simulink model "test"  (R2024b)
settings: Solver=FixedStepAuto  StartTime=0.0  StopTime=inf  FixedStep=0.01  RelTol=1e-3
undefined symbols (not defined in the file): DiscIntNeverNeededParam, LF
libraries: instrumentseriallib x11
settings Model: Creator=USER  LastModifiedBy=USER
settings OptimizationCC: DefaultParameterBehavior=Inlined  EnhancedBackFolding=on  PassReuseOutputArgsAs=Individual arguments  ZeroExternalMemoryAtStartup=off  ZeroInternalMemoryAtStartup=off  OptimizeBlockOrder=speed  DifferentSizesBufferReuse=on  OptimizationCustomize=off  EfficientTunableParamExpr=on
settings DebuggingCC: ParameterTunabilityLossMsg=error
settings SFSimCC: MATLABDynamicMemAlloc=off
settings RTWCC: Description=Embedded Coder  SystemTargetFile=ert.tlc  GenCodeOnly=on  TemplateMakefile=ert_default_tmf
settings CodeAppCC: ForceParamTrailComments=on  IgnoreCustomStorageClasses=off  OperatorAnnotations=on  SimulinkDataObjDesc=on  SFDataObjDesc=on  InsertBlockDesc=on
settings ERTTargetCC: TargetLangStandard=C99 (ISO)  GenerateSampleERTMain=on  ERTCustomFileTemplate=example_file_process.tlc

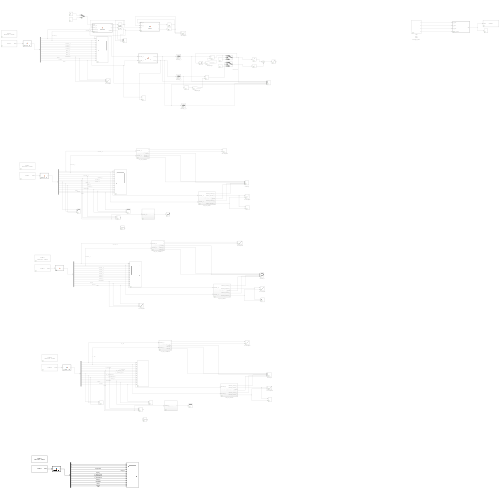
[thumbnail: Simulink's stored preview of the top-level diagram]
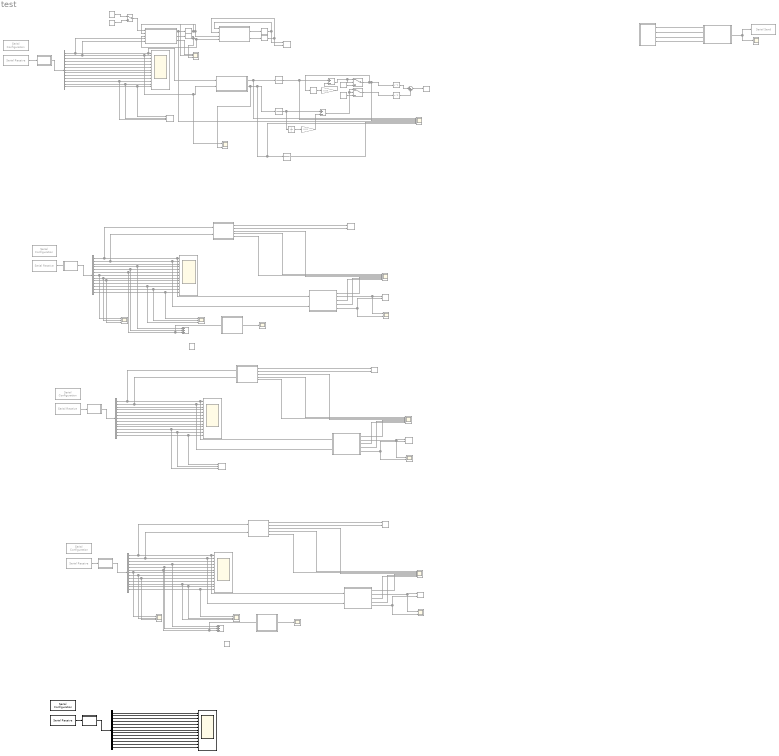
== system test ==
  1:Kp 2:Ki 3:Kd 4:target_pwm : Subsystem  Commented=on  mask{P_gain=1.0, I_gain=0.1, D_gain=0, PWM_speed=2000}
      mask prompts: P_gain "P gain"; I_gain "I gain"; D_gain "D gain"; PWM_speed "PWM Speed"
      mask DialogControl ParameterGroupVar Prompt: 파라미터
  Add : Sum  Commented=on  Inputs=+++
  Add1 : Sum  Commented=on  Inputs=+-
  Add2 : Sum  Commented=on  Inputs=+-
  Add3 : Sum  Commented=on  Inputs=+++
  Atan1 : Trigonometry  Commented=on  Operator=atan2
  Atan2 : Trigonometry  Commented=on  Operator=atan2
  Constant : Constant  Commented=on  Value=0
  Constant1 : Constant  Commented=on
  Constant3 : Constant  Commented=on  Value=0
  Constant4 : Constant  Commented=on  Value=0
  Demux{,1..3} (4 alike) : Demux  Commented=on  Outputs=13
  Demux4 : Demux  Outputs=13
  MATLAB Function : MATLAB Function  Commented=on  TreatAsAtomicUnit=on
  MATLAB Function1 : MATLAB Function  Commented=on  TreatAsAtomicUnit=on
  MATLAB Function2 : MATLAB Function  Commented=on  TreatAsAtomicUnit=on
  MATLAB Function3 : MATLAB Function  Commented=on  TreatAsAtomicUnit=on
  MATLAB Function4 : MATLAB Function  Commented=on  TreatAsAtomicUnit=on
  MATLAB Function5 : MATLAB Function  Commented=on  TreatAsAtomicUnit=on
  MATLAB Function6 : MATLAB Function  Commented=on  TreatAsAtomicUnit=on
  MATLAB Function7 : MATLAB Function  Commented=on  TreatAsAtomicUnit=on
  MATLAB Function8 : MATLAB Function  TreatAsAtomicUnit=on
  Manual Switch : ManualSwitch  Commented=on
  Memory{,1..4} (5 alike) : Memory  Commented=on
  Scope{,9..10,12,16} (5 alike) : Scope  Commented=on  NumInputPorts=3
  Scope1 : Scope  Commented=on
  Scope11 : Scope  Commented=on
  Scope13 : Scope  Commented=on
  Scope{4..5,7,14} (4 alike) : Scope  Commented=on  NumInputPorts=2
  Scope{2,6,8,15} (4 alike) : Scope  Commented=on  NumInputPorts=13
  Scope20 : Scope  NumInputPorts=13
  Scope3 : Scope  Commented=on  NumInputPorts=6
  Serial Configuration : instrumentseriallib/Serial Configuration  Priority=-200000  Commented=on  PortSel=COM17  Port=COM17  ComPort=COM17  BaudRate=115200  DataBits=8  Parity=none  StopBits=1  ByteOrder=big-endian  FlowControl=none  Timeout=1  SimulateUsing=Interpreted execution  BlockInModel=on  aMode=1
  Serial Configuration1 : instrumentseriallib/Serial Configuration  Priority=-200000  Commented=on  PortSel=COM17  Port=COM17  ComPort=COM17  BaudRate=115200  DataBits=8  Parity=none  StopBits=1  ByteOrder=big-endian  FlowControl=none  Timeout=1  SimulateUsing=Interpreted execution  BlockInModel=on  aMode=1
  Serial Configuration2 : instrumentseriallib/Serial Configuration  Priority=-200000  Commented=on  PortSel=COM17  Port=COM17  ComPort=COM17  BaudRate=115200  DataBits=8  Parity=none  StopBits=1  ByteOrder=big-endian  FlowControl=none  Timeout=1  SimulateUsing=Interpreted execution  BlockInModel=on  aMode=1
  Serial Configuration3 : instrumentseriallib/Serial Configuration  Priority=-200000  Commented=on  PortSel=COM19  Port=COM19  ComPort=COM19  BaudRate=115200  DataBits=8  Parity=none  StopBits=1  ByteOrder=big-endian  FlowControl=none  Timeout=1  SimulateUsing=Interpreted execution  BlockInModel=on  aMode=1
  Serial Configuration4 : instrumentseriallib/Serial Configuration  Priority=-200000  PortSel=COM19  Port=COM19  ComPort=COM19  BaudRate=115200  DataBits=8  Parity=none  StopBits=1  ByteOrder=big-endian  FlowControl=none  Timeout=1  SimulateUsing=Interpreted execution  BlockInModel=on  aMode=1
  Serial Receive : instrumentseriallib/Serial Receive  Priority=1  Commented=on  PortSel=COM17  Port=COM17  ComPort=COM17  DataType=uint8  SaveDataType=uint8  ToggleHeader=off  Header=[]  ToggleDataSize=on  DataSize=[1 130]  ToggleTerminator=on  Terminator=LF ('\n')  CustomTerminator=[]  InputFormat=Column major  EnableBlockingMode=on  ActionDataUnavailable=Output last received value  ActionWhenDataUnavailable=Output last received value  CustomValue=0  SampleTime=0.01  SimulateUsing=Interpreted execution  BlockInModel=on  aMode=1
  Serial Receive1 : instrumentseriallib/Serial Receive  Priority=1  Commented=on  PortSel=COM17  Port=COM17  ComPort=COM17  DataType=uint8  SaveDataType=uint8  ToggleHeader=off  Header=[]  ToggleDataSize=on  DataSize=[1 130]  ToggleTerminator=on  Terminator=LF ('\n')  CustomTerminator=[]  InputFormat=Column major  EnableBlockingMode=on  ActionDataUnavailable=Output last received value  ActionWhenDataUnavailable=Output last received value  CustomValue=0  SampleTime=0.01  SimulateUsing=Interpreted execution  BlockInModel=on  aMode=1
  Serial Receive2 : instrumentseriallib/Serial Receive  Priority=1  Commented=on  PortSel=COM17  Port=COM17  ComPort=COM17  DataType=uint8  SaveDataType=uint8  ToggleHeader=off  Header=[]  ToggleDataSize=on  DataSize=[1 130]  ToggleTerminator=on  Terminator=LF ('\n')  CustomTerminator=[]  InputFormat=Column major  EnableBlockingMode=on  ActionDataUnavailable=Output last received value  ActionWhenDataUnavailable=Output last received value  CustomValue=0  SampleTime=0.01  SimulateUsing=Interpreted execution  BlockInModel=on  aMode=1
  Serial Receive3 : instrumentseriallib/Serial Receive  Priority=1  Commented=on  PortSel=COM19  Port=COM19  ComPort=COM19  DataType=uint8  SaveDataType=uint8  ToggleHeader=off  Header=[]  ToggleDataSize=on  DataSize=[1 130]  ToggleTerminator=on  Terminator=LF ('\n')  CustomTerminator=[]  InputFormat=Column major  EnableBlockingMode=on  ActionDataUnavailable=Output last received value  ActionWhenDataUnavailable=Output last received value  CustomValue=0  SampleTime=0.01  SimulateUsing=Interpreted execution  BlockInModel=on  aMode=1
  Serial Receive4 : instrumentseriallib/Serial Receive  Priority=1  PortSel=COM19  Port=COM19  ComPort=COM19  DataType=uint8  SaveDataType=uint8  ToggleHeader=off  Header=[]  ToggleDataSize=on  DataSize=[1 130]  ToggleTerminator=on  Terminator=LF ('\n')  CustomTerminator=[]  InputFormat=Column major  EnableBlockingMode=on  ActionDataUnavailable=Output last received value  ActionWhenDataUnavailable=Output last received value  CustomValue=0  SampleTime=0.01  SimulateUsing=Interpreted execution  BlockInModel=on  aMode=1
  Serial Send : instrumentseriallib/Serial Send  Priority=1  Commented=on  PortSel=COM17  Port=COM17  ComPort=COM17  Header=[]  Terminator=<none>  CustomTerminator=[]  EnableBlockingMode=on  SimulateUsing=Interpreted execution  BlockInModel=on  aMode=1
  Sqrt : Sqrt  Commented=on
  Square : Math  Commented=on  Operator=square
  Square1 : Math  Commented=on  Operator=square
  Subsystem : Subsystem  Commented=on
  Subsystem1 : Subsystem  Commented=on
  Sum : Sum  Commented=on  Inputs=|++
  Switch : Switch  Commented=on  Criteria=u2 > Threshold  SaturateOnIntegerOverflow=off  InputSameDT=off
  Switch1 : Switch  Commented=on  Criteria=u2 > Threshold  SaturateOnIntegerOverflow=off  InputSameDT=off
  Unit Delay1 : UnitDelay  Commented=on  SampleTime=-1  HasFrameUpgradeWarning=on
  XY Graph{,1,5..7} (5 alike) : Record  Commented=on  FileSettingsInternal="{\"entries\":[{\"content\":{\"excelSettings\":{\"content\":{},\"type\":\"Streamout.ExcelSettings\"}},\"type\":\"Streamout.FileSettingStorage\",\"uuid\":\"\"}],\"packageUris\":[\"http:\\/\\/schema.mathworks.com\\/mf0\\/streamout_blocks\\/R2020a\"],\"version\":\"1.0\"}"  Layout=[1 1]  SignalsInternal="{\"entries\":[{\"content\":{},\"type\":\"RecordBlkView.InputSignals\",\"uuid\":\"\"}],\"packageUris\":[\"http:\\/\\/schema.mathworks.com\\/mf0\\/streamout_blocks\\/R2020a\"],\"version\":\"1.0\"}"  VisualizationBindings="{\"xyplotplugin\":{\"info\":[{\"series\":[],\"subplotID\":1}]}}"  CompatibilityTag=XY
  XY Graph2 : Record  Commented=on  FileSettingsInternal="{\"entries\":[{\"content\":{\"excelSettings\":{\"content\":{},\"type\":\"Streamout.ExcelSettings\"}},\"type\":\"Streamout.FileSettingStorage\",\"uuid\":\"\"}],\"packageUris\":[\"http:\\/\\/schema.mathworks.com\\/mf0\\/streamout_blocks\\/R2020a\"],\"version\":\"1.0\"}"  Layout=[1 1]  SignalsInternal="{\"entries\":[{\"content\":{\"signals\":[{\"content\":{\"blockPath\":[],\"dimensions\":[1],\"domain\":\"\",\"lineColor\":\"#edb120\",\"lineWidth\":2,\"port\":1,\"signalID\":1,\"signalName\":\"vel_loc_nofilter:1\"},\"type\":\"RecordBlkView.Signal\",\"uuid\":\"\"},{\"content\":{\"blockPath\":[],\"dimensions\":[1],\"domain\":\"\",\"lineColor\":\"#7e2f8e\",\"lineWidth\":2,\"port\":2,\"signalID\":2,\"signalName\":\"vel_loc_nofilter:2\"},\"type\":\"RecordBlkView.Signal\",\"uuid\":\"\"}]},\"type\":\"RecordBlkView.InputSignals\",\"uuid\":\"\"}],\"packageUris\":[\"http:\\/\\/schema.mathworks.com\\/mf0\\/streamout_blocks\\/R2020a\"],\"version\":\"1.0\"}"  VisualizationBindings="{\"xyplotplugin\":{\"info\":[{\"series\":[],\"subplotID\":1}]}}"  CompatibilityTag=XY
  XY Graph3 : Record  Commented=on  FileSettingsInternal="{\"entries\":[{\"content\":{\"excelSettings\":{\"content\":{},\"type\":\"Streamout.ExcelSettings\"}},\"type\":\"Streamout.FileSettingStorage\",\"uuid\":\"\"}],\"packageUris\":[\"http:\\/\\/schema.mathworks.com\\/mf0\\/streamout_blocks\\/R2020a\"],\"version\":\"1.0\"}"  Layout=[1 1]  SignalsInternal="{\"entries\":[{\"content\":{\"signals\":[{\"content\":{\"blockPath\":[],\"dimensions\":[1],\"domain\":\"\",\"lineColor\":\"#64d413\",\"lineWidth\":2,\"port\":1,\"signalID\":1,\"signalName\":\"vel_loc_nofilter2:1\"},\"type\":\"RecordBlkView.Signal\",\"uuid\":\"\"},{\"content\":{\"blockPath\":[],\"dimensions\":[1],\"domain\":\"\",\"lineColor\":\"#ff13a6\",\"lineWidth\":2,\"port\":2,\"signalID\":2,\"signalName\":\"vel_loc_nofilter2:2\"},\"type\":\"RecordBlkView.Signal\",\"uuid\":\"\"}]},\"type\":\"RecordBlkView.InputSignals\",\"uuid\":\"\"}],\"packageUris\":[\"http:\\/\\/schema.mathworks.com\\/mf0\\/streamout_blocks\\/R2020a\"],\"version\":\"1.0\"}"  VisualizationBindings="{\"xyplotplugin\":{\"info\":[{\"series\":[],\"subplotID\":1}]}}"  CompatibilityTag=XY
  XY Graph4 : Record  Commented=on  FileSettingsInternal="{\"entries\":[{\"content\":{\"excelSettings\":{\"content\":{},\"type\":\"Streamout.ExcelSettings\"}},\"type\":\"Streamout.FileSettingStorage\",\"uuid\":\"\"}],\"packageUris\":[\"http:\\/\\/schema.mathworks.com\\/mf0\\/streamout_blocks\\/R2020a\"],\"version\":\"1.0\"}"  Layout=[1 1]  SignalsInternal="{\"entries\":[{\"content\":{\"signals\":[{\"content\":{\"blockPath\":[],\"dimensions\":[1],\"domain\":\"\",\"lineColor\":\"#77ac30\",\"lineWidth\":2,\"port\":1,\"signalID\":1,\"signalName\":\"vel_loc_Filter:2\"},\"type\":\"RecordBlkView.Signal\",\"uuid\":\"\"},{\"content\":{\"blockPath\":[],\"dimensions\":[1],\"domain\":\"\",\"lineColor\":\"#4dbeee\",\"lineWidth\":2,\"port\":2,\"signalID\":2,\"signalName\":\"vel_loc_Filter:5\"},\"type\":\"RecordBlkView.Signal\",\"uuid\":\"\"}]},\"type\":\"RecordBlkView.InputSignals\",\"uuid\":\"\"}],\"packageUris\":[\"http:\\/\\/schema.mathworks.com\\/mf0\\/streamout_blocks\\/R2020a\"],\"version\":\"1.0\"}"  VisualizationBindings="{\"xyplotplugin\":{\"info\":[{\"series\":[],\"subplotID\":1}]}}"  CompatibilityTag=XY
  XY Graph8 : Record  Commented=on  FileSettingsInternal="{\"entries\":[{\"content\":{\"excelSettings\":{\"content\":{},\"type\":\"Streamout.ExcelSettings\"}},\"type\":\"Streamout.FileSettingStorage\",\"uuid\":\"\"}],\"packageUris\":[\"http:\\/\\/schema.mathworks.com\\/mf0\\/streamout_blocks\\/R2020a\"],\"version\":\"1.0\"}"  Layout=[1 1]  SignalsInternal="{\"entries\":[{\"content\":{\"signals\":[{\"content\":{\"blockPath\":[],\"dimensions\":[1],\"domain\":\"\",\"lineColor\":\"#fe330a\",\"lineWidth\":2,\"port\":1,\"signalID\":1,\"signalName\":\"vel_loc_Filter2:2\"},\"type\":\"RecordBlkView.Signal\",\"uuid\":\"\"},{\"content\":{\"blockPath\":[],\"dimensions\":[1],\"domain\":\"\",\"lineColor\":\"#22b573\",\"lineWidth\":2,\"port\":2,\"signalID\":2,\"signalName\":\"vel_loc_Filter2:5\"},\"type\":\"RecordBlkView.Signal\",\"uuid\":\"\"}]},\"type\":\"RecordBlkView.InputSignals\",\"uuid\":\"\"}],\"packageUris\":[\"http:\\/\\/schema.mathworks.com\\/mf0\\/streamout_blocks\\/R2020a\"],\"version\":\"1.0\"}"  VisualizationBindings="{\"xyplotplugin\":{\"info\":[{\"series\":[],\"subplotID\":1}]}}"  CompatibilityTag=XY
  damping1 : Gain  Commented=on  Gain=0.05
  damping2 : Gain  Commented=on  Gain=0.01
  vel_loc_Filter : Subsystem  Commented=on
  vel_loc_Filter1 : Subsystem  Commented=on
  vel_loc_Filter2 : Subsystem  Commented=on
  vel_loc_nofilter : Subsystem  Commented=on
  vel_loc_nofilter1 : Subsystem  Commented=on
  vel_loc_nofilter2 : Subsystem  Commented=on
  velocity : Scope  Commented=on  NumInputPorts=6
  velocity1 : Scope  Commented=on  NumInputPorts=6
  velocity2 : Scope  Commented=on  NumInputPorts=6
  velocity_x : DiscreteIntegrator  Commented=on  IntegratorMethod=Integration: Backward Euler  gainval=0.01  InitialCondition=0.001  SampleTime=0.01  ICPrevOutput=DiscIntNeverNeededParam  ICPrevScaledInput=DiscIntNeverNeededParam
  velocity_y : DiscreteIntegrator  Commented=on  IntegratorMethod=Integration: Backward Euler  gainval=0.01  SampleTime=0.01  ICPrevOutput=DiscIntNeverNeededParam  ICPrevScaledInput=DiscIntNeverNeededParam
  velocity_y1 : DiscreteIntegrator  Commented=on  IntegratorMethod=Integration: Backward Euler  gainval=0.01  InitialCondition=0.001  SampleTime=0.01  ICPrevOutput=DiscIntNeverNeededParam  ICPrevScaledInput=DiscIntNeverNeededParam
  wires:
  Serial Receive/1 -> MATLAB Function/1(u)
  1:Kp 2:Ki 3:Kd 4:target_pwm/4(Out4) -> MATLAB Function1/4(pwm_speed)
  1:Kp 2:Ki 3:Kd 4:target_pwm/1(Out1) -> MATLAB Function1/1(p_gain)
  1:Kp 2:Ki 3:Kd 4:target_pwm/2(Out2) -> MATLAB Function1/2(i_gain)
  1:Kp 2:Ki 3:Kd 4:target_pwm/3(Out3) -> MATLAB Function1/3(d_gain)
  MATLAB Function1/1(out) -> Scope1/1, Serial Send/1
  MATLAB Function/1(y) -> Demux/1
  Demux/1 -> MATLAB Function2/4(ACCEL_X), MATLAB Function4/1(ACCEL_X), Scope2/1  "ACCEL_X"
  Demux/2 -> MATLAB Function2/5(ACCEL_Y), Scope4/1, MATLAB Function4/2(ACCEL_Y), Scope2/2  "ACCEL_Y"
  Demux/3 -> Scope2/3  "ACCEL_Z"
  Demux/4 -> Scope2/4  "GYRO_X"
  Demux/5 -> Scope2/5  "GYRO_Y"
  Demux/6 -> Scope2/6  "GYRO_Z"
  Demux/7 -> Scope2/7  "MAG_X"
  Demux/8 -> Scope2/8  "MAG_Y"
  Demux/9 -> Scope2/9  "MAG_Z"
  MATLAB Function2/1(vx) -> Scope3/4, Memory/1
  Memory/1 -> Scope/2, MATLAB Function3/3(vx), MATLAB Function2/2(prev_vx)
  MATLAB Function2/2(vy) -> Memory1/1
  Memory1/1 -> Scope/3, MATLAB Function3/4(vy), MATLAB Function2/3(prev_vy)
  MATLAB Function3/1(x) -> Memory2/1
  MATLAB Function3/2(y) -> Memory3/1
  Memory2/1 -> XY Graph/1, MATLAB Function3/1(prev_x)
  Memory3/1 -> XY Graph/2, MATLAB Function3/2(prev_y)
  MATLAB Function2/3(speed) -> Scope/1
  Manual Switch/1 -> MATLAB Function2/1(stop)
  Constant/1 -> Manual Switch/1
  Constant1/1 -> Manual Switch/2
  Demux/11 -> XY Graph1/3, Scope2/11  "ROLL"
  Demux/12 -> XY Graph1/2, Scope2/12  "PITCH"
  Demux/13 -> XY Graph1/1, Scope2/13  "YAW"
  Demux/10 -> Scope2/10  "HEADING"
  MATLAB Function4/1(accel_x) -> velocity_x/1, Scope3/1
  MATLAB Function4/2(accel_y) -> Scope4/2, Scope3/6, velocity_y1/1, velocity_y/1
  Square/1 -> Sum/1
  Square1/1 -> Sum/2
  Sum/1 -> Sqrt/1
  velocity_y/1 -> Add2/1, Unit Delay1/1
  velocity_x/1 -> Add1/1, Scope3/2
  Constant3/1 -> Switch/3
  Switch/1 -> Memory4/1, Square/1, Scope3/3  "filter and d"
  Add2/1 -> Switch1/1, Switch1/2
  Constant4/1 -> Switch1/3
  Switch1/1 -> Square1/1
  Unit Delay1/1 -> damping2/1
  damping2/1 -> Add2/2
  Memory4/1 -> damping1/1
  damping1/1 -> Add1/2
  Add1/1 -> Switch/2, Switch/1
  velocity_y1/1 -> Scope3/5
  Demux1/9 -> Scope10/3, Scope6/9  "MAG_Z"
  Demux1/8 -> Scope10/2, Scope6/8  "MAG_Y"
  Demux1/3 -> Scope6/3  "ACCEL_Z"
  Demux1/4 -> Add/1, Scope6/4  "GYRO_X"
  Serial Receive1/1 -> MATLAB Function5/1(u)
  Demux1/1 -> vel_loc_nofilter/1(ACCEL_X), vel_loc_Filter/1(ACCEL_X), Scope6/1  "ACCEL_X"
  Demux1/5 -> Add/2, Scope6/5  "GYRO_Y"
  Demux1/11 -> Scope9/3, Scope6/11  "ROLL"
  Demux1/13 -> Scope9/1, Scope6/13  "YAW"
  Demux1/6 -> Subsystem/1(GYRO_Z), Add/3, Scope6/6  "GYRO_Z"
  Demux1/7 -> Scope10/1, Scope6/7  "MAG_X"
  Demux1/10 -> Scope6/10  "HEADING"
  MATLAB Function5/1(y) -> Demux1/1
  Demux1/12 -> Scope9/2, Scope6/12  "PITCH"
  Demux1/2 -> vel_loc_nofilter/2(ACCEL_Y), vel_loc_Filter/2(ACCEL_Y), Scope6/2  "ACCEL_Y"
  vel_loc_nofilter/1(x) -> XY Graph2/1
  vel_loc_nofilter/2(y) -> XY Graph2/2
  vel_loc_nofilter/4(velocity_x) -> velocity/1
  vel_loc_nofilter/5(velocity_y) -> velocity/2
  vel_loc_nofilter/3(velocity) -> velocity/3
  vel_loc_Filter/1(filtered_velocity_x) -> velocity/4
  vel_loc_Filter/4(filtered_velocity_y) -> velocity/5
  vel_loc_Filter/3(speed) -> velocity/6
  vel_loc_Filter/2(filtered_location_x) -> Scope5/1, XY Graph4/1
  vel_loc_Filter/5(filtered_location_y) -> XY Graph4/2, Scope5/2
  vel_loc_nofilter1/3(velocity) -> velocity1/3
  Demux2/2 -> vel_loc_nofilter1/2(ACCEL_Y), vel_loc_Filter1/2(ACCEL_Y), Scope8/2  "ACCEL_Y"
  vel_loc_nofilter1/1(x) -> XY Graph5/1
  MATLAB Function6/1(y) -> Demux2/1
  Demux2/10 -> Scope8/10  "HEADING"
  Demux2/6 -> Scope8/6  "GYRO_Z"
  Demux2/7 -> Scope8/7  "MAG_X"
  Demux2/11 -> XY Graph6/3, Scope8/11  "ROLL"
  Demux2/1 -> vel_loc_nofilter1/1(ACCEL_X), vel_loc_Filter1/1(ACCEL_X), Scope8/1  "ACCEL_X"
  Serial Receive2/1 -> MATLAB Function6/1(u)
  Demux2/9 -> Scope8/9  "MAG_Z"
  Demux2/3 -> Scope8/3  "ACCEL_Z"
  Demux2/8 -> Scope8/8  "MAG_Y"
  vel_loc_nofilter1/2(y) -> XY Graph5/2
  Demux2/12 -> XY Graph6/2, Scope8/12  "PITCH"
  Demux2/13 -> XY Graph6/1, Scope8/13  "YAW"
  vel_loc_Filter1/3(speed) -> velocity1/6
  vel_loc_nofilter1/5(velocity_y) -> velocity1/2
  Demux2/4 -> Scope8/4  "GYRO_X"
  vel_loc_nofilter1/4(velocity_x) -> velocity1/1
  vel_loc_Filter1/2(filtered_location_x) -> Scope7/1, XY Graph7/1
  vel_loc_Filter1/1(filtered_velocity_x) -> velocity1/4
  Demux2/5 -> Scope8/5  "GYRO_Y"
  vel_loc_Filter1/5(filtered_location_y) -> XY Graph7/2, Scope7/2
  vel_loc_Filter1/4(filtered_velocity_y) -> velocity1/5
  Subsystem/1(Out1) -> Scope11/1
  vel_loc_nofilter2/2(y) -> XY Graph3/2
  Demux3/2 -> vel_loc_nofilter2/2(ACCEL_Y), vel_loc_Filter2/2(ACCEL_Y), Scope15/2  "L_dis"
  vel_loc_nofilter2/1(x) -> XY Graph3/1
  vel_loc_Filter2/3(speed) -> velocity2/6
  Demux3/13 -> Scope16/1, Scope15/13  "YAW"
  Demux3/11 -> Scope16/3, Scope15/11  "ROLL"
  vel_loc_nofilter2/3(velocity) -> velocity2/3
  Demux3/6 -> Subsystem1/1(GYRO_Z), Add3/3, Scope15/6  "L_parking_spot"
  Demux3/3 -> Scope15/3  "R_obstacle"
  Demux3/5 -> Add3/2, Scope15/5  "R_parking_spot"
  Demux3/10 -> Scope15/10  "HEADING"
  Demux3/1 -> vel_loc_nofilter2/1(ACCEL_X), vel_loc_Filter2/1(ACCEL_X), Scope15/1  "R_dis"
  Demux3/4 -> Add3/1, Scope15/4  "L_Obstacle"
  vel_loc_Filter2/1(filtered_velocity_x) -> velocity2/4
  Demux3/9 -> Scope12/3, Scope15/9  "MAG_Z"
  Serial Receive3/1 -> MATLAB Function7/1(u)
  Demux3/7 -> Scope12/1, Scope15/7  "R_spotdistacne"
  vel_loc_Filter2/2(filtered_location_x) -> Scope14/1, XY Graph8/1
  vel_loc_nofilter2/4(velocity_x) -> velocity2/1
  Demux3/12 -> Scope16/2, Scope15/12  "PITCH"
  vel_loc_Filter2/4(filtered_velocity_y) -> velocity2/5
  Demux3/8 -> Scope12/2, Scope15/8  "L_spotdistacne"
  vel_loc_nofilter2/5(velocity_y) -> velocity2/2
  vel_loc_Filter2/5(filtered_location_y) -> XY Graph8/2, Scope14/2
  Subsystem1/1(Out1) -> Scope13/1
  MATLAB Function7/1(y) -> Demux3/1
  Demux4/2 -> Scope20/2  "y"
  Serial Receive4/1 -> MATLAB Function8/1(u)
  Demux4/8 -> Scope20/8  "L_spotdistacne"
  MATLAB Function8/1(y) -> Demux4/1
  Demux4/5 -> Scope20/5  "target_y"
  Demux4/3 -> Scope20/3  "waypointidx"
  Demux4/10 -> Scope20/10  "HEADING"
  Demux4/11 -> Scope20/11  "ROLL"
  Demux4/13 -> Scope20/13  "YAW"
  Demux4/1 -> Scope20/1  "x"
  Demux4/4 -> Scope20/4  "target_x"
  Demux4/12 -> Scope20/12  "PITCH"
  Demux4/7 -> Scope20/7  "R_spotdistacne"
  Demux4/9 -> Scope20/9  "MAG_Z"
  Demux4/6 -> Scope20/6  "L_parking_spot"

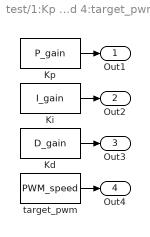
== system test/1:Kp 2:Ki 3:Kd 4:target_pwm ==
  Kd : Constant  Value=D_gain
  Ki : Constant  Value=I_gain
  Kp : Constant  Value=P_gain
  target_pwm : Constant  Value=PWM_speed
  Out1 : Outport
  Out2 : Outport  Port=2
  Out3 : Outport  Port=3
  Out4 : Outport  Port=4
  wires:
  Kd/1 -> Out3/1
  Kp/1 -> Out1/1
  Ki/1 -> Out2/1
  target_pwm/1 -> Out4/1

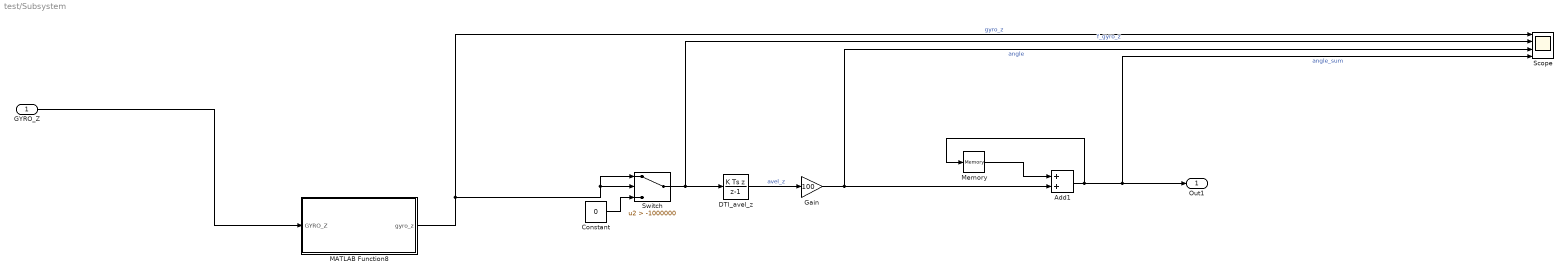
== system test/Subsystem ==
  GYRO_Z : Inport
  Add1 : Sum
  Constant : Constant  Value=0
  DTI_avel_z : DiscreteIntegrator  IntegratorMethod=Integration: Backward Euler  gainval=0.01  SampleTime=0.01  ICPrevOutput=DiscIntNeverNeededParam  ICPrevScaledInput=DiscIntNeverNeededParam
  Gain : Gain  Gain=100
  MATLAB Function8 : MATLAB Function  TreatAsAtomicUnit=on
  Memory : Memory
  Scope : Scope  NumInputPorts=4
  Switch : Switch  Criteria=u2 > Threshold  Threshold=-1000000  SaturateOnIntegerOverflow=off  InputSameDT=off
  Out1 : Outport
  wires:
  GYRO_Z/1 -> MATLAB Function8/1(GYRO_Z)
  MATLAB Function8/1(gyro_z) -> Scope/1, Switch/1, Switch/2  "gyro_z"
  Gain/1 -> Scope/3, Add1/2  "angle"
  Constant/1 -> Switch/3
  Switch/1 -> Scope/2, DTI_avel_z/1  "f_gyro_z"
  DTI_avel_z/1 -> Gain/1  "avel_z"
  Add1/1 -> Scope/4, Out1/1, Memory/1  "angle_sum"
  Memory/1 -> Add1/1

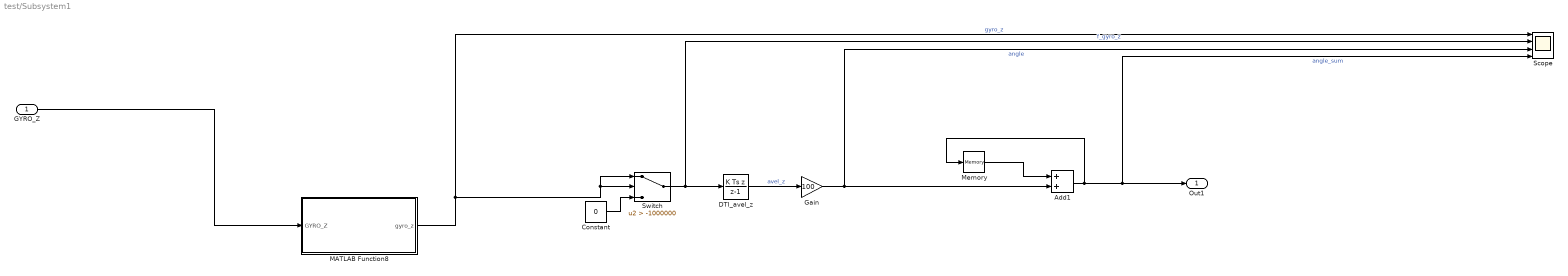
== system test/Subsystem1 ==
  GYRO_Z : Inport
  Add1 : Sum
  Constant : Constant  Value=0
  DTI_avel_z : DiscreteIntegrator  IntegratorMethod=Integration: Backward Euler  gainval=0.01  SampleTime=0.01  ICPrevOutput=DiscIntNeverNeededParam  ICPrevScaledInput=DiscIntNeverNeededParam
  Gain : Gain  Gain=100
  MATLAB Function8 : MATLAB Function  TreatAsAtomicUnit=on
  Memory : Memory
  Scope : Scope  NumInputPorts=4
  Switch : Switch  Criteria=u2 > Threshold  Threshold=-1000000  SaturateOnIntegerOverflow=off  InputSameDT=off
  Out1 : Outport
  wires:
  GYRO_Z/1 -> MATLAB Function8/1(GYRO_Z)
  MATLAB Function8/1(gyro_z) -> Scope/1, Switch/1, Switch/2  "gyro_z"
  Gain/1 -> Scope/3, Add1/2  "angle"
  Constant/1 -> Switch/3
  Switch/1 -> Scope/2, DTI_avel_z/1  "f_gyro_z"
  DTI_avel_z/1 -> Gain/1  "avel_z"
  Add1/1 -> Scope/4, Out1/1, Memory/1  "angle_sum"
  Memory/1 -> Add1/1

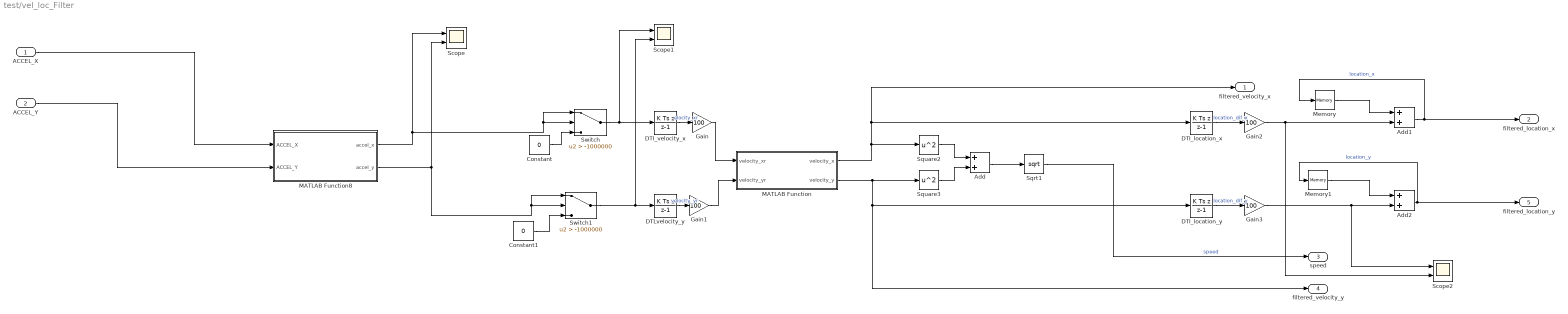
== system test/vel_loc_Filter ==
  ACCEL_X : Inport
  ACCEL_Y : Inport  Port=2
  Add : Sum
  Add1 : Sum
  Add2 : Sum
  Constant : Constant  Value=0
  Constant1 : Constant  Value=0
  DTI_location_x : DiscreteIntegrator  IntegratorMethod=Integration: Backward Euler  gainval=0.01  SampleTime=0.01  ICPrevOutput=DiscIntNeverNeededParam  ICPrevScaledInput=DiscIntNeverNeededParam
  DTI_location_y : DiscreteIntegrator  IntegratorMethod=Integration: Backward Euler  gainval=0.01  SampleTime=0.01  ICPrevOutput=DiscIntNeverNeededParam  ICPrevScaledInput=DiscIntNeverNeededParam
  DTI_velocity_x : DiscreteIntegrator  IntegratorMethod=Integration: Backward Euler  gainval=0.01  SampleTime=0.01  ICPrevOutput=DiscIntNeverNeededParam  ICPrevScaledInput=DiscIntNeverNeededParam
  DTLvelocity_y : DiscreteIntegrator  IntegratorMethod=Integration: Backward Euler  gainval=0.01  SampleTime=0.01  ICPrevOutput=DiscIntNeverNeededParam  ICPrevScaledInput=DiscIntNeverNeededParam
  Gain{,1..3} (4 alike) : Gain  Gain=100
  MATLAB Function : MATLAB Function  TreatAsAtomicUnit=on
  MATLAB Function8 : MATLAB Function  TreatAsAtomicUnit=on
  Memory : Memory
  Memory1 : Memory
  Scope : Scope  NumInputPorts=2
  Scope1 : Scope  NumInputPorts=2
  Scope2 : Scope  NumInputPorts=2
  Sqrt1 : Sqrt
  Square2 : Math  Operator=square
  Square3 : Math  Operator=square
  Switch : Switch  Criteria=u2 > Threshold  Threshold=-1000000  SaturateOnIntegerOverflow=off  InputSameDT=off
  Switch1 : Switch  Criteria=u2 > Threshold  Threshold=-1000000  SaturateOnIntegerOverflow=off  InputSameDT=off
  filtered_velocity_x : Outport
  filtered_location_x : Outport  Port=2
  speed : Outport  Port=3
  filtered_velocity_y : Outport  Port=4
  filtered_location_y : Outport  Port=5
  wires:
  DTLvelocity_y/1 -> Gain1/1  "velocity_yr"
  Add/1 -> Sqrt1/1
  DTI_velocity_x/1 -> Gain/1  "elocity_xr"
  Square3/1 -> Add/2
  MATLAB Function8/2(accel_y) -> Switch1/1, Switch1/2, Scope/2
  MATLAB Function8/1(accel_x) -> Scope/1, Switch/1, Switch/2
  Square2/1 -> Add/1
  Sqrt1/1 -> speed/1  "speed"
  ACCEL_X/1 -> MATLAB Function8/1(ACCEL_X)
  ACCEL_Y/1 -> MATLAB Function8/2(ACCEL_Y)
  DTI_location_x/1 -> Gain2/1  "location_dif_x"
  Memory/1 -> Add1/1
  Add1/1 -> Memory/1, filtered_location_x/1  "location_x"
  Add2/1 -> filtered_location_y/1, Memory1/1  "location_y"
  Memory1/1 -> Add2/1
  DTI_location_y/1 -> Gain3/1  "location_dif_y"
  Switch/1 -> Scope1/1, DTI_velocity_x/1
  Switch1/1 -> Scope1/2, DTLvelocity_y/1
  Constant1/1 -> Switch1/3
  Constant/1 -> Switch/3
  MATLAB Function/1(velocity_x) -> Square2/1, DTI_location_x/1, filtered_velocity_x/1
  MATLAB Function/2(velocity_y) -> Square3/1, DTI_location_y/1, filtered_velocity_y/1
  Gain/1 -> MATLAB Function/1(velocity_xr)
  Gain1/1 -> MATLAB Function/2(velocity_yr)
  Gain2/1 -> Scope2/2, Add1/2
  Gain3/1 -> Scope2/1, Add2/2

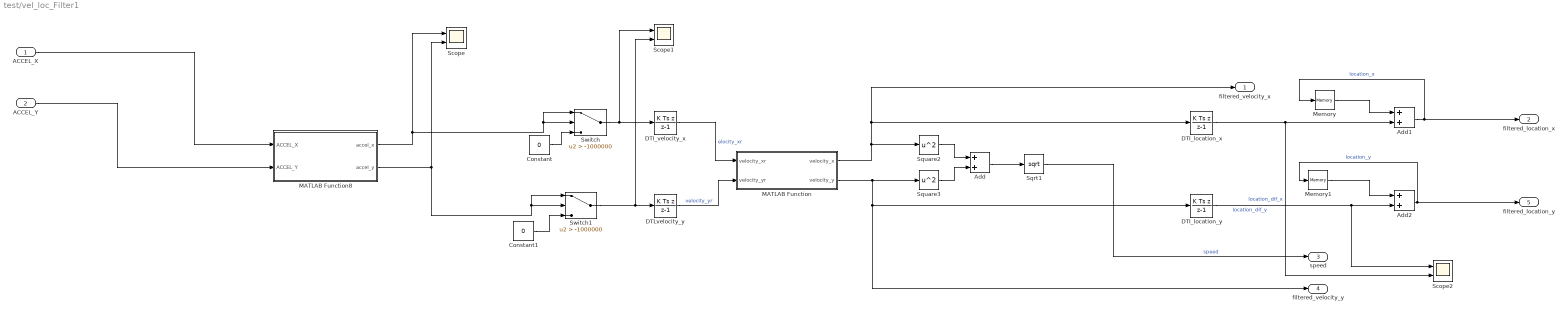
== system test/vel_loc_Filter1 ==
  ACCEL_X : Inport
  ACCEL_Y : Inport  Port=2
  Add : Sum
  Add1 : Sum
  Add2 : Sum
  Constant : Constant  Value=0
  Constant1 : Constant  Value=0
  DTI_location_x : DiscreteIntegrator  IntegratorMethod=Integration: Backward Euler  gainval=0.01  SampleTime=0.01  ICPrevOutput=DiscIntNeverNeededParam  ICPrevScaledInput=DiscIntNeverNeededParam
  DTI_location_y : DiscreteIntegrator  IntegratorMethod=Integration: Backward Euler  gainval=0.01  SampleTime=0.01  ICPrevOutput=DiscIntNeverNeededParam  ICPrevScaledInput=DiscIntNeverNeededParam
  DTI_velocity_x : DiscreteIntegrator  IntegratorMethod=Integration: Backward Euler  gainval=0.01  SampleTime=0.01  ICPrevOutput=DiscIntNeverNeededParam  ICPrevScaledInput=DiscIntNeverNeededParam
  DTLvelocity_y : DiscreteIntegrator  IntegratorMethod=Integration: Backward Euler  gainval=0.01  SampleTime=0.01  ICPrevOutput=DiscIntNeverNeededParam  ICPrevScaledInput=DiscIntNeverNeededParam
  MATLAB Function : MATLAB Function  TreatAsAtomicUnit=on
  MATLAB Function8 : MATLAB Function  TreatAsAtomicUnit=on
  Memory : Memory
  Memory1 : Memory
  Scope : Scope  NumInputPorts=2
  Scope1 : Scope  NumInputPorts=2
  Scope2 : Scope  NumInputPorts=2
  Sqrt1 : Sqrt
  Square2 : Math  Operator=square
  Square3 : Math  Operator=square
  Switch : Switch  Criteria=u2 > Threshold  Threshold=-1000000  SaturateOnIntegerOverflow=off  InputSameDT=off
  Switch1 : Switch  Criteria=u2 > Threshold  Threshold=-1000000  SaturateOnIntegerOverflow=off  InputSameDT=off
  filtered_velocity_x : Outport
  filtered_location_x : Outport  Port=2
  speed : Outport  Port=3
  filtered_velocity_y : Outport  Port=4
  filtered_location_y : Outport  Port=5
  wires:
  DTLvelocity_y/1 -> MATLAB Function/2(velocity_yr)  "velocity_yr"
  Add/1 -> Sqrt1/1
  DTI_velocity_x/1 -> MATLAB Function/1(velocity_xr)  "elocity_xr"
  Square3/1 -> Add/2
  MATLAB Function8/2(accel_y) -> Switch1/1, Switch1/2, Scope/2
  MATLAB Function8/1(accel_x) -> Scope/1, Switch/1, Switch/2
  Square2/1 -> Add/1
  Sqrt1/1 -> speed/1  "speed"
  ACCEL_X/1 -> MATLAB Function8/1(ACCEL_X)
  ACCEL_Y/1 -> MATLAB Function8/2(ACCEL_Y)
  DTI_location_x/1 -> Scope2/2, Add1/2  "location_dif_x"
  Memory/1 -> Add1/1
  Add1/1 -> Memory/1, filtered_location_x/1  "location_x"
  Add2/1 -> filtered_location_y/1, Memory1/1  "location_y"
  Memory1/1 -> Add2/1
  DTI_location_y/1 -> Scope2/1, Add2/2  "location_dif_y"
  Switch/1 -> Scope1/1, DTI_velocity_x/1
  Switch1/1 -> Scope1/2, DTLvelocity_y/1
  Constant1/1 -> Switch1/3
  Constant/1 -> Switch/3
  MATLAB Function/1(velocity_x) -> Square2/1, DTI_location_x/1, filtered_velocity_x/1
  MATLAB Function/2(velocity_y) -> Square3/1, DTI_location_y/1, filtered_velocity_y/1

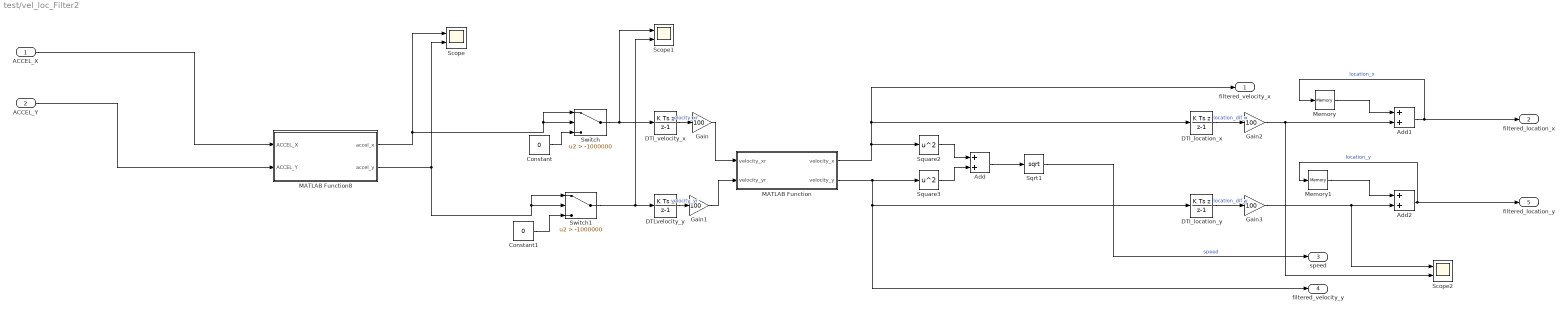
== system test/vel_loc_Filter2 ==
  ACCEL_X : Inport
  ACCEL_Y : Inport  Port=2
  Add : Sum
  Add1 : Sum
  Add2 : Sum
  Constant : Constant  Value=0
  Constant1 : Constant  Value=0
  DTI_location_x : DiscreteIntegrator  IntegratorMethod=Integration: Backward Euler  gainval=0.01  SampleTime=0.01  ICPrevOutput=DiscIntNeverNeededParam  ICPrevScaledInput=DiscIntNeverNeededParam
  DTI_location_y : DiscreteIntegrator  IntegratorMethod=Integration: Backward Euler  gainval=0.01  SampleTime=0.01  ICPrevOutput=DiscIntNeverNeededParam  ICPrevScaledInput=DiscIntNeverNeededParam
  DTI_velocity_x : DiscreteIntegrator  IntegratorMethod=Integration: Backward Euler  gainval=0.01  SampleTime=0.01  ICPrevOutput=DiscIntNeverNeededParam  ICPrevScaledInput=DiscIntNeverNeededParam
  DTLvelocity_y : DiscreteIntegrator  IntegratorMethod=Integration: Backward Euler  gainval=0.01  SampleTime=0.01  ICPrevOutput=DiscIntNeverNeededParam  ICPrevScaledInput=DiscIntNeverNeededParam
  Gain{,1..3} (4 alike) : Gain  Gain=100
  MATLAB Function : MATLAB Function  TreatAsAtomicUnit=on
  MATLAB Function8 : MATLAB Function  TreatAsAtomicUnit=on
  Memory : Memory
  Memory1 : Memory
  Scope : Scope  NumInputPorts=2
  Scope1 : Scope  NumInputPorts=2
  Scope2 : Scope  NumInputPorts=2
  Sqrt1 : Sqrt
  Square2 : Math  Operator=square
  Square3 : Math  Operator=square
  Switch : Switch  Criteria=u2 > Threshold  Threshold=-1000000  SaturateOnIntegerOverflow=off  InputSameDT=off
  Switch1 : Switch  Criteria=u2 > Threshold  Threshold=-1000000  SaturateOnIntegerOverflow=off  InputSameDT=off
  filtered_velocity_x : Outport
  filtered_location_x : Outport  Port=2
  speed : Outport  Port=3
  filtered_velocity_y : Outport  Port=4
  filtered_location_y : Outport  Port=5
  wires:
  DTLvelocity_y/1 -> Gain1/1  "velocity_yr"
  Add/1 -> Sqrt1/1
  DTI_velocity_x/1 -> Gain/1  "elocity_xr"
  Square3/1 -> Add/2
  MATLAB Function8/2(accel_y) -> Switch1/1, Switch1/2, Scope/2
  MATLAB Function8/1(accel_x) -> Scope/1, Switch/1, Switch/2
  Square2/1 -> Add/1
  Sqrt1/1 -> speed/1  "speed"
  ACCEL_X/1 -> MATLAB Function8/1(ACCEL_X)
  ACCEL_Y/1 -> MATLAB Function8/2(ACCEL_Y)
  DTI_location_x/1 -> Gain2/1  "location_dif_x"
  Memory/1 -> Add1/1
  Add1/1 -> Memory/1, filtered_location_x/1  "location_x"
  Add2/1 -> filtered_location_y/1, Memory1/1  "location_y"
  Memory1/1 -> Add2/1
  DTI_location_y/1 -> Gain3/1  "location_dif_y"
  Switch/1 -> Scope1/1, DTI_velocity_x/1
  Switch1/1 -> Scope1/2, DTLvelocity_y/1
  Constant1/1 -> Switch1/3
  Constant/1 -> Switch/3
  MATLAB Function/1(velocity_x) -> Square2/1, DTI_location_x/1, filtered_velocity_x/1
  MATLAB Function/2(velocity_y) -> Square3/1, DTI_location_y/1, filtered_velocity_y/1
  Gain/1 -> MATLAB Function/1(velocity_xr)
  Gain1/1 -> MATLAB Function/2(velocity_yr)
  Gain2/1 -> Scope2/2, Add1/2
  Gain3/1 -> Scope2/1, Add2/2

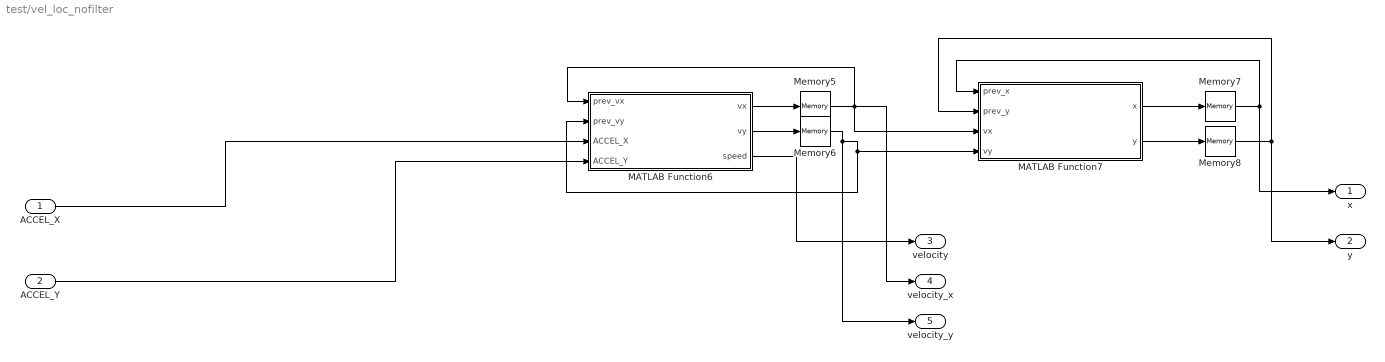
== system test/vel_loc_nofilter ==
  ACCEL_X : Inport
  ACCEL_Y : Inport  Port=2
  MATLAB Function6 : MATLAB Function  TreatAsAtomicUnit=on
  MATLAB Function7 : MATLAB Function  TreatAsAtomicUnit=on
  Memory{5..8} (4 alike) : Memory
  x : Outport
  y : Outport  Port=2
  velocity : Outport  Port=3
  velocity_x : Outport  Port=4
  velocity_y : Outport  Port=5
  wires:
  Memory6/1 -> velocity_y/1, MATLAB Function7/4(vy), MATLAB Function6/2(prev_vy)
  Memory8/1 -> y/1, MATLAB Function7/2(prev_y)
  MATLAB Function6/2(vy) -> Memory6/1
  MATLAB Function6/1(vx) -> Memory5/1
  Memory5/1 -> velocity_x/1, MATLAB Function7/3(vx), MATLAB Function6/1(prev_vx)
  MATLAB Function7/1(x) -> Memory7/1
  Memory7/1 -> x/1, MATLAB Function7/1(prev_x)
  MATLAB Function7/2(y) -> Memory8/1
  ACCEL_Y/1 -> MATLAB Function6/4(ACCEL_Y)
  ACCEL_X/1 -> MATLAB Function6/3(ACCEL_X)
  MATLAB Function6/3(speed) -> velocity/1

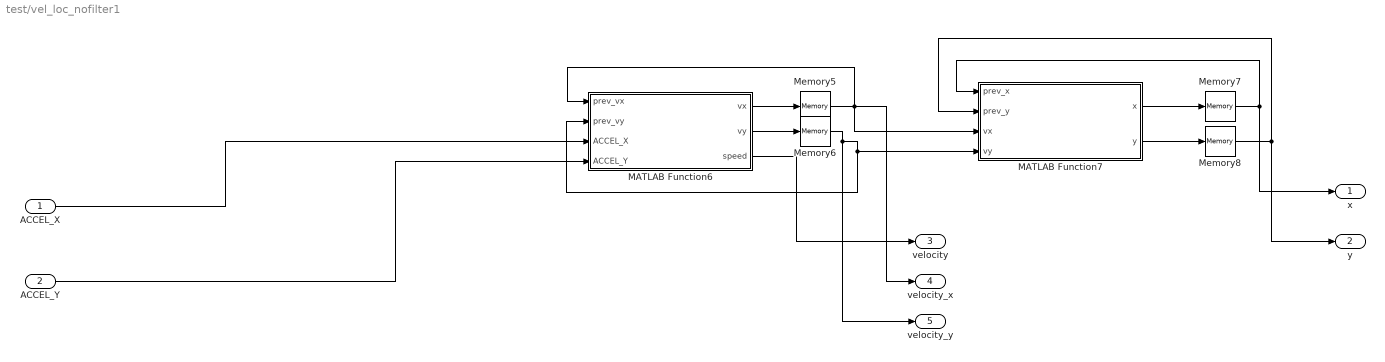
== system test/vel_loc_nofilter1 ==
  ACCEL_X : Inport
  ACCEL_Y : Inport  Port=2
  MATLAB Function6 : MATLAB Function  TreatAsAtomicUnit=on
  MATLAB Function7 : MATLAB Function  TreatAsAtomicUnit=on
  Memory{5..8} (4 alike) : Memory
  x : Outport
  y : Outport  Port=2
  velocity : Outport  Port=3
  velocity_x : Outport  Port=4
  velocity_y : Outport  Port=5
  wires:
  Memory6/1 -> velocity_y/1, MATLAB Function7/4(vy), MATLAB Function6/2(prev_vy)
  Memory8/1 -> y/1, MATLAB Function7/2(prev_y)
  MATLAB Function6/2(vy) -> Memory6/1
  MATLAB Function6/1(vx) -> Memory5/1
  Memory5/1 -> velocity_x/1, MATLAB Function7/3(vx), MATLAB Function6/1(prev_vx)
  MATLAB Function7/1(x) -> Memory7/1
  Memory7/1 -> x/1, MATLAB Function7/1(prev_x)
  MATLAB Function7/2(y) -> Memory8/1
  ACCEL_Y/1 -> MATLAB Function6/4(ACCEL_Y)
  ACCEL_X/1 -> MATLAB Function6/3(ACCEL_X)
  MATLAB Function6/3(speed) -> velocity/1

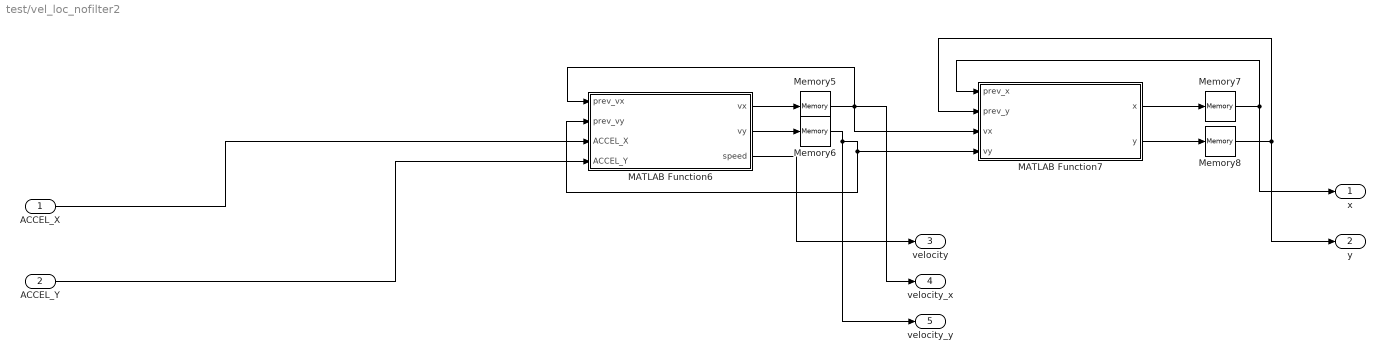
== system test/vel_loc_nofilter2 ==
  ACCEL_X : Inport
  ACCEL_Y : Inport  Port=2
  MATLAB Function6 : MATLAB Function  TreatAsAtomicUnit=on
  MATLAB Function7 : MATLAB Function  TreatAsAtomicUnit=on
  Memory{5..8} (4 alike) : Memory
  x : Outport
  y : Outport  Port=2
  velocity : Outport  Port=3
  velocity_x : Outport  Port=4
  velocity_y : Outport  Port=5
  wires:
  Memory6/1 -> velocity_y/1, MATLAB Function7/4(vy), MATLAB Function6/2(prev_vy)
  Memory8/1 -> y/1, MATLAB Function7/2(prev_y)
  MATLAB Function6/2(vy) -> Memory6/1
  MATLAB Function6/1(vx) -> Memory5/1
  Memory5/1 -> velocity_x/1, MATLAB Function7/3(vx), MATLAB Function6/1(prev_vx)
  MATLAB Function7/1(x) -> Memory7/1
  Memory7/1 -> x/1, MATLAB Function7/1(prev_x)
  MATLAB Function7/2(y) -> Memory8/1
  ACCEL_Y/1 -> MATLAB Function6/4(ACCEL_Y)
  ACCEL_X/1 -> MATLAB Function6/3(ACCEL_X)
  MATLAB Function6/3(speed) -> velocity/1

== matlab function test/vel_loc_Filter/MATLAB Function ==
  data: velocity_xr input; velocity_x output; velocity_y output; velocity_yr input
function [velocity_x, velocity_y] = vel_noise(velocity_xr, velocity_yr)
    
    velocity_x = velocity_xr;
    velocity_y = velocity_yr;
    if(velocity_xr<0.02 && velocity_xr>-0.02)
        velocity_x=0;
    end
    if(velocity_yr<0.02 && velocity_yr>-0.02)
        velocity_y=0;
    end
end

== matlab function test/MATLAB Function6 ==
  data: u input; y output
function y = parsing_all(u)
    u_double = double(u); % 입력 문자의 ASCII 값
    digits = u_double - 48; % ASCII '0'(48)을 빼서 숫자로 변환

    n = length(digits);
    num_values = n / 10; % 10개씩 데이터 분할
    y = zeros(1, num_values, 'double');

    for i = 1:num_values
        start_idx = (i - 1) * 10 + 1;
        end_idx = start_idx + 8;

        % 숫자 값 검증 (0~9 범위를 벗어나면 오류 처리)
        %if any(digits(start_idx:end_idx) > 9 | digits(start_idx:end_idx) < 0)
        %    error('Invalid digit found in input data!');
        %end

        % 숫자 변환
        data = int64(0);
        for a = 0:8
            data = data + int64(digits(end_idx - a)) * int64(10)^a;
        end

        % 부호 판별 ('m'이면 음수)
        if u(start_idx + 9) == 'm'
            data = -data;
        end

        % double(float)로 변환
        y(i) = double(data) / 1000.0;
    end
end

== matlab function test/vel_loc_Filter1/MATLAB Function ==
  data: velocity_xr input; velocity_x output; velocity_y output; velocity_yr input
function [velocity_x, velocity_y] = vel_noise(velocity_xr, velocity_yr)
    
    velocity_x = velocity_xr;
    velocity_y = velocity_yr;
    if(velocity_xr<0.02 && velocity_xr>-0.02)
        velocity_x=0;
    end
    if(velocity_yr<0.02 && velocity_yr>-0.02)
        velocity_y=0;
    end
end

== matlab function test/vel_loc_Filter1/MATLAB Function8 ==
  data: ACCEL_X input; accel_x output; ACCEL_Y input; accel_y output
function [accel_x, accel_y] = findspeed(ACCEL_X, ACCEL_Y)

    accel_x=ACCEL_X;
    accel_y=ACCEL_Y;
    threshold = 0.02; % 노이즈
    if abs(accel_x) < threshold && abs(accel_x) > -threshold 
        accel_x = 0;
    end
    if abs(accel_y) < threshold && abs(accel_y) > -threshold 
        accel_y = 0;
    end
    accel_x = accel_x * 981; % g -> cm/s^2
    accel_y = accel_y * 981;

    %if abs(accel_x) >10000000 || abs(accel_x) <10000000 
    %    accel_x = 0;
    %end
    %if abs(accel_y) >10000000 || abs(accel_y) <10000000 
    %    accel_y = 0;
    %end
end

== matlab function test/vel_loc_nofilter1/MATLAB Function6 ==
  data: prev_vx input; prev_vy input; ACCEL_X input; vx output; ACCEL_Y input; vy output; speed output
function [vx, vy, speed] = findspeed(prev_vx, prev_vy, ACCEL_X, ACCEL_Y)
    dt = 0.01;
    threshold = 0.02; % 노이즈
    if abs(ACCEL_X) < threshold
        ACCEL_X = 0;
    end
    if abs(ACCEL_Y) < threshold
        ACCEL_Y = 0;
    end

    ACCEL_X = ACCEL_X * 981; % g -> cm/s^2
    ACCEL_Y = ACCEL_Y * 981;

    vx = prev_vx + ACCEL_X * dt;
    vy = prev_vy + ACCEL_Y * dt;
    speed = sqrt(vx^2 + vy^2 );
end

== matlab function test/vel_loc_nofilter1/MATLAB Function7 ==
  data: prev_x input; prev_y input; vx input; vy input; x output; y output
function [x, y] = findloc(prev_x, prev_y, vx, vy)
    dt = 0.01; 

    % 위치 업데이트 (적분 1회 더 진행)
    x = prev_x + vx * dt;
    y = prev_y + vy * dt;
end

== matlab function test/MATLAB Function1 ==
  data: p_gain input; out output; i_gain input; d_gain input; pwm_speed input
function out = dataScaling(p_gain, i_gain, d_gain, pwm_speed)
    % 데이터 스케일링
    p_uint16 = uint16(p_gain * 1000);
    i_uint16 = uint16(i_gain * 1000);
    d_uint16 = uint16(d_gain * 1000);
    pwm_uint16 = uint16(pwm_speed + 5000);
    
    % 각 uint16 값을 상위/하위 바이트로 분리
    p_high = uint8(bitshift(p_uint16, -8));
    p_low = uint8(bitand(p_uint16, 255));
    
    i_high = uint8(bitshift(i_uint16, -8));
    i_low = uint8(bitand(i_uint16, 255));
    
    d_high = uint8(bitshift(d_uint16, -8));
    d_low = uint8(bitand(d_uint16, 255));
    
    pwm_high = uint8(bitshift(pwm_uint16, -8));
    pwm_low = uint8(bitand(pwm_uint16, 255));
    
    % 전송할 순서대로 바이트 배열 구성
    out = [p_high; p_low; i_high; i_low; d_high; d_low; pwm_high; pwm_low];
end

== matlab function test/MATLAB Function7 ==
  data: u input; y output
function y = parsing_all(u)
    u_double = double(u); % 입력 문자의 ASCII 값
    digits = u_double - 48; % ASCII '0'(48)을 빼서 숫자로 변환

    n = length(digits);
    num_values = n / 10; % 10개씩 데이터 분할
    y = zeros(1, num_values, 'double');

    for i = 1:num_values
        start_idx = (i - 1) * 10 + 1;
        end_idx = start_idx + 8;

        % 숫자 값 검증 (0~9 범위를 벗어나면 오류 처리)
        %if any(digits(start_idx:end_idx) > 9 | digits(start_idx:end_idx) < 0)
        %    error('Invalid digit found in input data!');
        %end

        % 숫자 변환
        data = int64(0);
        for a = 0:8
            data = data + int64(digits(end_idx - a)) * int64(10)^a;
        end

        % 부호 판별 ('m'이면 음수)
        if u(start_idx + 9) == 'm'
            data = -data;
        end

        % double(float)로 변환
        y(i) = double(data) / 1000.0;
    end
end

== matlab function test/Subsystem/MATLAB Function8 ==
  data: GYRO_Z input; gyro_z output
function gyro_z  = findspeed(GYRO_Z)

    gyro_z=GYRO_Z;
    
    threshold = 0.6; % 노이즈
    if abs(gyro_z) < threshold && abs(gyro_z) > -threshold 
        gyro_z = 0;
    end

end

== matlab function test/Subsystem1/MATLAB Function8 ==
  data: GYRO_Z input; gyro_z output
function gyro_z  = findspeed(GYRO_Z)

    gyro_z=GYRO_Z;
    
    threshold = 0.6; % 노이즈
    if abs(gyro_z) < threshold && abs(gyro_z) > -threshold 
        gyro_z = 0;
    end

end

== matlab function test/vel_loc_Filter2/MATLAB Function ==
  data: velocity_xr input; velocity_x output; velocity_y output; velocity_yr input
function [velocity_x, velocity_y] = vel_noise(velocity_xr, velocity_yr)
    
    velocity_x = velocity_xr;
    velocity_y = velocity_yr;
    if(velocity_xr<0.02 && velocity_xr>-0.02)
        velocity_x=0;
    end
    if(velocity_yr<0.02 && velocity_yr>-0.02)
        velocity_y=0;
    end
end

== matlab function test/vel_loc_Filter2/MATLAB Function8 ==
  data: ACCEL_X input; accel_x output; ACCEL_Y input; accel_y output
function [accel_x, accel_y] = findspeed(ACCEL_X, ACCEL_Y)

    accel_x=ACCEL_X;
    accel_y=ACCEL_Y;
    threshold = 0.02; % 노이즈
    if abs(accel_x) < threshold && abs(accel_x) > -threshold 
        accel_x = 0;
    end
    if abs(accel_y) < threshold && abs(accel_y) > -threshold 
        accel_y = 0;
    end
    accel_x = accel_x * 981; % g -> cm/s^2
    accel_y = accel_y * 981;

    %if abs(accel_x) >10000000 || abs(accel_x) <10000000 
    %    accel_x = 0;
    %end
    %if abs(accel_y) >10000000 || abs(accel_y) <10000000 
    %    accel_y = 0;
    %end
end

== matlab function test/vel_loc_nofilter2/MATLAB Function6 ==
  data: prev_vx input; prev_vy input; ACCEL_X input; vx output; ACCEL_Y input; vy output; speed output
function [vx, vy, speed] = findspeed(prev_vx, prev_vy, ACCEL_X, ACCEL_Y)
    dt = 0.01;
    threshold = 0.02; % 노이즈
    if abs(ACCEL_X) < threshold
        ACCEL_X = 0;
    end
    if abs(ACCEL_Y) < threshold
        ACCEL_Y = 0;
    end

    ACCEL_X = ACCEL_X * 981; % g -> cm/s^2
    ACCEL_Y = ACCEL_Y * 981;

    vx = prev_vx + ACCEL_X * dt;
    vy = prev_vy + ACCEL_Y * dt;
    speed = sqrt(vx^2 + vy^2 );
end

== matlab function test/vel_loc_nofilter2/MATLAB Function7 ==
  data: prev_x input; prev_y input; vx input; vy input; x output; y output
function [x, y] = findloc(prev_x, prev_y, vx, vy)
    dt = 0.01; 

    % 위치 업데이트 (적분 1회 더 진행)
    x = prev_x + vx * dt;
    y = prev_y + vy * dt;
end

== matlab function test/MATLAB Function8 ==
  data: u input; y output
function y = parsing_all(u)
    u_double = double(u); % 입력 문자의 ASCII 값
    digits = u_double - 48; % ASCII '0'(48)을 빼서 숫자로 변환

    n = length(digits);
    num_values = n / 10; % 10개씩 데이터 분할
    y = zeros(1, num_values, 'double');

    for i = 1:num_values
        start_idx = (i - 1) * 10 + 1;
        end_idx = start_idx + 8;

        % 숫자 값 검증 (0~9 범위를 벗어나면 오류 처리)
        %if any(digits(start_idx:end_idx) > 9 | digits(start_idx:end_idx) < 0)
        %    error('Invalid digit found in input data!');
        %end

        % 숫자 변환
        data = int64(0);
        for a = 0:8
            data = data + int64(digits(end_idx - a)) * int64(10)^a;
        end

        % 부호 판별 ('m'이면 음수)
        if u(start_idx + 9) == 'm'
            data = -data;
        end

        % double(float)로 변환
        y(i) = double(data) / 1000.0;
    end
end

== matlab function test/MATLAB Function ==
  data: u input; y output
function y = parsing_all(u)
    u_double = double(u); % 문자를 숫자로 변환 (ASCII 코드 기준)
    digits = double(u_double - 48); % ASCII '0'의 값(48)을 빼서 실제 숫자로 변환
    n = length(digits); % 입력 데이터 길이 확인

    num_values = n / 10; % 10개씩 다른 정보 저장됨
    y = zeros(1, num_values, 'double'); % 결과 배열을 double로 생성 (float 결과 보장)

    for i = 1:num_values
        start_idx = (i - 1) * 10 + 1; % 시작 위치
        end_idx = start_idx + 8; % 숫자 9자리 (부호 제외)

        data = int64(0); % 정수형으로 초기화 (오버플로우 방지)
        for a = 0:8 % 9자리 숫자 변환
            data = data + int64(digits(end_idx - a)) * int64(10)^a;
        end

        % 부호 확인 ('m'이면 음수, 'p'이면 양수)
        if (digits(start_idx + 9) == (uint8('m') - 48))
            data = -data;
        end

        % 결과를 double(float)로 변환
        y(i) = double(data) / 10000.0;  % 4자리 소수점 변환 (예제)
    end
end

== matlab function test/MATLAB Function2 ==
  data: stop input; prev_vx input; prev_vy input; ACCEL_X input; vx output; ACCEL_Y input; vy output; speed output
function [vx, vy, speed] = findspeed(stop, prev_vx, prev_vy, ACCEL_X, ACCEL_Y)
    dt = 0.01;
    vx=0;
    vy=0;
    speed=0;
    if(stop==0)  %진행중(모터 돌아감)
        threshold = 0.02; % 노이즈
        if abs(ACCEL_X) < threshold
            ACCEL_X = 0;
        end
        if abs(ACCEL_Y) < threshold
            ACCEL_Y = 0;
        end

        ACCEL_X = ACCEL_X * 981; % g -> cm/s^2
        ACCEL_Y = ACCEL_Y * 981;
    
        vx = prev_vx + ACCEL_X * dt;
        vy = prev_vy + ACCEL_Y * dt;
        speed = sqrt(vx^2 + vy^2 );
    end
    if(stop==1) %차량 정지
        vx = 0;
        vy = 0;
        speed=0;
    end   
end

== matlab function test/MATLAB Function3 ==
  data: prev_x input; prev_y input; vx input; vy input; x output; y output
function [x, y] = findloc(prev_x, prev_y, vx, vy)
    dt = 0.01; 

    % 위치 업데이트 (적분 1회 더 진행)
    x = prev_x + vx * dt;
    y = prev_y + vy * dt;
end

== matlab function test/MATLAB Function4 ==
  data: ACCEL_X input; accel_x output; ACCEL_Y input; accel_y output
function [accel_x, accel_y] = findspeed(ACCEL_X, ACCEL_Y)

    accel_x=ACCEL_X;
    accel_y=ACCEL_Y;
    threshold = 0.02; % 노이즈
    if abs(accel_x) < threshold && abs(accel_x) > -threshold 
        accel_x = 0;
    end
    if abs(accel_y) < threshold && abs(accel_y) > -threshold 
        accel_y = 0;
    end
    %if abs(accel_x) >10000 || abs(accel_x) <10000 
    %    accel_x = 0;
    %end
    %if abs(accel_y) >10000 || abs(accel_y) <10000 
    %    accel_y = 0;
    %end
   % accel_x = accel_x * 981; % g -> cm/s^2
    %accel_y = accel_y * 981;
end

== matlab function test/MATLAB Function5 ==
  data: u input; y output
function y = parsing_all(u)
    u_double = double(u); % 입력 문자의 ASCII 값
    digits = u_double - 48; % ASCII '0'(48)을 빼서 숫자로 변환

    n = length(digits);
    num_values = n / 10; % 10개씩 데이터 분할
    y = zeros(1, num_values, 'double');

    for i = 1:num_values
        start_idx = (i - 1) * 10 + 1;
        end_idx = start_idx + 8;

        % 숫자 값 검증 (0~9 범위를 벗어나면 오류 처리)
        %if any(digits(start_idx:end_idx) > 9 | digits(start_idx:end_idx) < 0)
        %    error('Invalid digit found in input data!');
        %end

        % 숫자 변환
        data = int64(0);
        for a = 0:8
            data = data + int64(digits(end_idx - a)) * int64(10)^a;
        end

        % 부호 판별 ('m'이면 음수)
        if u(start_idx + 9) == 'm'
            data = -data;
        end

        % double(float)로 변환
        y(i) = double(data) / 1000.0;
    end
end

== matlab function test/vel_loc_nofilter/MATLAB Function6 ==
  data: prev_vx input; prev_vy input; ACCEL_X input; vx output; ACCEL_Y input; vy output; speed output
function [vx, vy, speed] = findspeed(prev_vx, prev_vy, ACCEL_X, ACCEL_Y)
    dt = 0.01;
    threshold = 0.02; % 노이즈
    if abs(ACCEL_X) < threshold
        ACCEL_X = 0;
    end
    if abs(ACCEL_Y) < threshold
        ACCEL_Y = 0;
    end

    ACCEL_X = ACCEL_X * 981; % g -> cm/s^2
    ACCEL_Y = ACCEL_Y * 981;

    vx = prev_vx + ACCEL_X * dt;
    vy = prev_vy + ACCEL_Y * dt;
    speed = sqrt(vx^2 + vy^2 );
end

== matlab function test/vel_loc_nofilter/MATLAB Function7 ==
  data: prev_x input; prev_y input; vx input; vy input; x output; y output
function [x, y] = findloc(prev_x, prev_y, vx, vy)
    dt = 0.01; 

    % 위치 업데이트 (적분 1회 더 진행)
    x = prev_x + vx * dt;
    y = prev_y + vy * dt;
end

== matlab function test/vel_loc_Filter/MATLAB Function8 ==
  data: ACCEL_X input; accel_x output; ACCEL_Y input; accel_y output
function [accel_x, accel_y] = findspeed(ACCEL_X, ACCEL_Y)

    accel_x=ACCEL_X;
    accel_y=ACCEL_Y;
    threshold = 0.02; % 노이즈
    if abs(accel_x) < threshold && abs(accel_x) > -threshold 
        accel_x = 0;
    end
    if abs(accel_y) < threshold && abs(accel_y) > -threshold 
        accel_y = 0;
    end
    accel_x = accel_x * 981; % g -> cm/s^2
    accel_y = accel_y * 981;

    %if abs(accel_x) >10000000 || abs(accel_x) <10000000 
    %    accel_x = 0;
    %end
    %if abs(accel_y) >10000000 || abs(accel_y) <10000000 
    %    accel_y = 0;
    %end
end
